simulink model "QC_pid_HIL_control"  (Simulink 7.4)
settings: Solver=ode45  StartTime=0.0  StopTime=inf  RelTol=1e-3
PreLoadFcn:
  | run quadrocopter_param
values from neighbouring files (symbols this model uses):
  phi0 = 0.15    [Quadrocopter_control_Driver.m]    (also in calc_stability.m = 0)
  r_phi0 = 0    [Quadrocopter_control_Driver.m]    (also in calc_stability.m)
  r_psi0 = 0    [Quadrocopter_control_Driver.m]    (also in calc_stability.m)
  r_theta0 = 0    [Quadrocopter_control_Driver.m]    (also in calc_stability.m)
  theta0 = 0.15    [Quadrocopter_control_Driver.m]    (also in calc_stability.m = 0)
  Ts = 0.01    [Reglerauslegung.m]    (also in Test_Reglerauslegung.m)
undefined symbols (not defined in the file or in its folder): boom, f1, f2, f3, f4, f5, g, I_x, I_y, I_z, m
libraries: Copter_Library x6, simulink x4, Control_lib x2
CloseFcn:
  | rtwprivate ssgensfun ModelCloseRequest QC_pid_HIL_control
settings Model: Creator=roczit00  LastModifiedBy=dsatikid

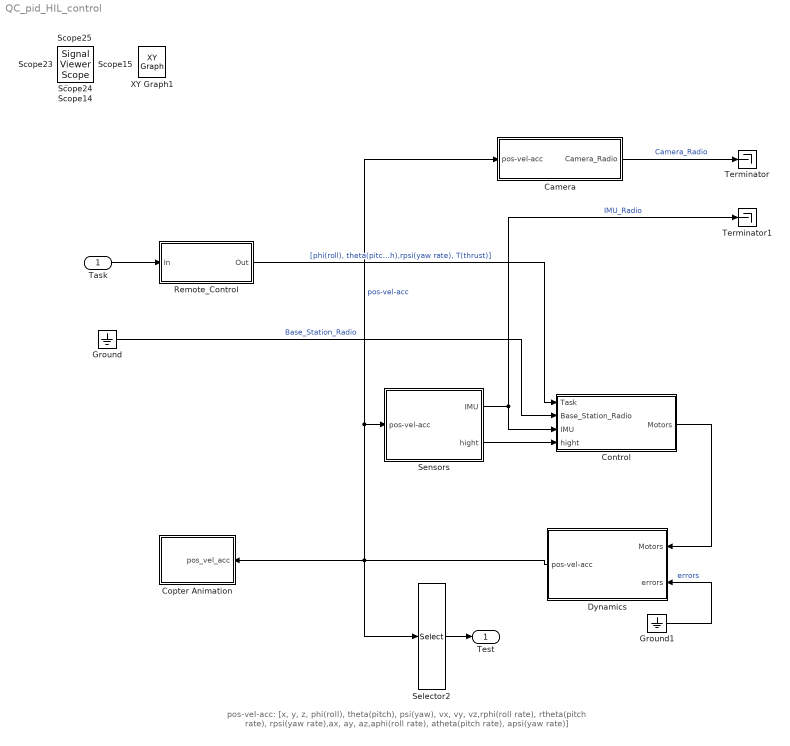
== system QC_pid_HIL_control ==
  note: pos-vel-acc: [x, y, z, phi(roll), theta(pitch), psi(yaw), vx, vy, vz,rphi(roll rate), rtheta(pitch rate), rpsi(yaw rate),ax, ay, az,aphi(roll rate), atheta(pitch rate), apsi(yaw rate)]
  Task : Inport  PortDimensions=4  OutDataType=fixdt(1, 16)  OutScaling=2^0
  Camera : Subsystem
  Control : Subsystem
  Copter Animation : Subsystem  mask(Quadrocopter Animation){AXES=[-100 100 -100 100 0 100], T_INT=1/25, K_VAR=Feste Position, K_POS=[10 0 2], K_ANGLE=27, A_ON=on, u_phi=on, u_theta=on, u_psi=on, u_x=on, u_y=on, u_z=off}
      mask prompts: AXES "Achsen Grenzen [xmin xmax ymin ymax zmin zmax]"; T_INT "Zeitintervall zwischen Aktualisierungen [s]:"; K_VAR "Kamera Art:"; K_POS "Ort der Kamera [xc yc zc]:"; K_ANGLE "Öffnungswinkel der Kamera [Grad]:"; A_ON "Animation Einschalten:"; u_phi "Use Input phi:"; u_theta "Use Input theta:"; u_psi "Use Input psi:"; u_x "Use Input x:"; u_y "Use Input y:"; u_z "Use Input z:"
      mask help: Erstellt eine 3-D animierte Ansicht eines Quadrocopters.
      mask init:
      | Config.axes = AXES;
      | Config.update = T_INT;
      | Config.camera_view = K_VAR;
      | Config.camera_pos = K_POS;
      | Config.view = K_ANGLE;
      | Config.Animenable = A_ON;
      | Config.phi = u_phi;
      | Config.theta = u_theta;
      | Config.psi = u_psi;
      | Config.x = u_x;
      | Config.y = u_y;
      | Config.z = u_z;
      mask Help:
      | <p>Dieser Block erstellt ein 3 dimensionales Fenster eines Quadrocopters.
      | 
      | <p><H4>Block Eingänge</H4>
      | Der Eingangsvektor bestehend aus:
      | <ul>
      | <li>X-Koordinate - Ort bezogen auf die X-Achse
      | <li>Y-Koordinate - Ort bezogen auf die Y-Achse
      | <li>Z-Koordinate - Ort bezogen auf die Z-Achse
      | <li>Psi - Yaw Drehung um die Z-Achse
      | <li>Phi - Roll Drehen um die Achse in Flugrichtung
      | <li>theta - pitch Neigung in Flugrichtung nach oben bzw. unten
      | </ul></p>
      mask StyleString: edit,edit,popup(Feste Position|Frei bewegbar),edit,edit,checkbox,checkbox,checkbox,checkbox,checkbox,checkbox,checkbox
  Dynamics : Subsystem
  Ground : Ground
  Ground1 : Ground
  Remote_Control : Subsystem
  Selector2 : Selector  InputPortWidth=19  IndexOptions=Index vector (dialog)  Indices=[4 5 6]  OutputSizes=1
  Sensors : Subsystem
  Terminator : Terminator
  Terminator1 : Terminator
  Test : Outport  OutDataType=fixdt(1, 16)  OutScaling=2^0
  Scope : SignalViewerScope  IOType=viewer  RefreshTime=0.035000
      settings: YMin=-12500  YMax=22500
  Scope11 : SignalViewerScope  IOType=viewer  LegendLocations="247.3333           139            72      20.33333"  RefreshTime=0.103216
      settings: ShowLegends=on  YMin=-1  YMax=0.75  SaveName=ScopeData11
  Scope14 : SignalViewerScope  IOType=viewer  ZoomMode=yonly  LegendLocations="236.3333           142            82      20.33333"  RefreshTime=0.148000
      settings: ShowLegends=on  YMin=-0.2  YMax=0.8  SaveName=ScopeData14
  Scope15 : SignalViewerScope  IOType=viewer  ZoomMode=yonly  LegendLocations="245.3333           139            74      20.33333"  RefreshTime=0.035000
      settings: ShowLegends=on  YMin=-50  YMax=30  SaveName=ScopeData15
  Scope23 : SignalViewerScope  IOType=viewer  LegendLocations="230.3333           178            71      20.33333"  RefreshTime=0.035000
      settings: ShowLegends=on  YMin=-2  YMax=0.25  SaveName=ScopeData23
  Scope24 : SignalViewerScope  IOType=viewer  LegendLocations="248.3333           141            75      20.33333"  RefreshTime=0.035000
      settings: ShowLegends=on  YMin=-0.3  YMax=0.3  SaveName=ScopeData24
  Scope25 : SignalViewerScope  IOType=viewer  LegendLocations="224.3333           129            85      25.33333"  RefreshTime=0.035000
      settings: ShowLegends=on  YMin=-0.05  YMax=0.175  SaveName=ScopeData25
  XY Graph1 : simulink/Sinks/XY Graph  IOType=viewer  SystemSampleTime=-1  xmin=-50  xmax=50  ymin=-50  ymax=50  st=Ts
  wires:
  Sensors/1(IMU) -> Terminator1/1, Control/3(IMU)  "IMU_Radio"
  Sensors/2(hight) -> Control/4(hight)
  Ground1/1 -> Dynamics/2(errors)  "errors"
  Control/1(Motors) -> Dynamics/1(Motors)
  Dynamics/1(pos-vel-acc) -> Sensors/1(pos-vel-acc), Camera/1(pos-vel-acc), Selector2/1, Copter Animation/1(pos_vel_acc)  "pos-vel-acc"
  Camera/1(Camera_Radio) -> Terminator/1  "Camera_Radio"
  Ground/1 -> Control/2(Base_Station_Radio)  "Base_Station_Radio"
  Remote_Control/1(Out) -> Control/1(Task)  "[phi(roll), theta(pitch),rpsi(yaw rate), T(thrust)]"
  Selector2/1 -> Test/1
  Task/1 -> Remote_Control/1(In)

== system QC_pid_HIL_control/Camera ==
  pos-vel-acc : Inport  OutDataType=fixdt(1, 16)  OutScaling=2^0
  Camera_Radio : Outport  OutDataType=fixdt(1, 16)  OutScaling=2^0
  wires:
  pos-vel-acc/1 -> Camera_Radio/1

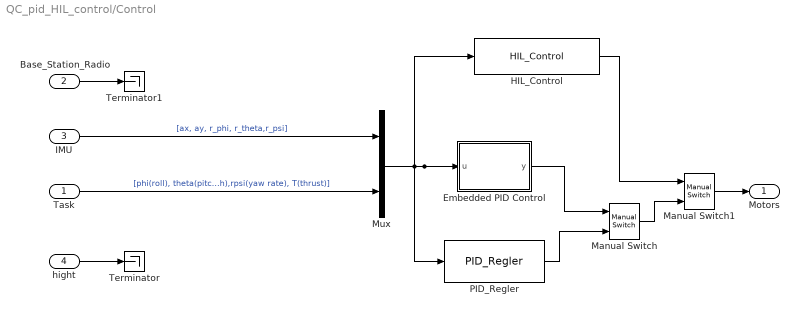
== system QC_pid_HIL_control/Control ==
  Task : Inport  PortDimensions=4  DataType=double  OutDataType=fixdt(1, 16)  OutScaling=2^0  OutDataTypeStr=double
  Base_Station_Radio : Inport  Port=2  OutDataType=fixdt(1, 16)  OutScaling=2^0
  IMU : Inport  Port=3  OutDataType=fixdt(1, 16)  OutScaling=2^0
  hight : Inport  Port=4  DataType=int16  OutDataType=fixdt(1, 16)  OutScaling=2^0  OutDataTypeStr=int16
  Embedded PID Control : Stateflow chart
  HIL_Control : Control_lib/HIL_Control  enabled=on
  Manual Switch : simulink/Signal Routing/Manual Switch  SystemSampleTime=-1  sw=0  action=0  varsize=off
  Manual Switch1 : simulink/Signal Routing/Manual Switch  SystemSampleTime=-1  sw=1  action=0  varsize=off
  Mux : Mux  Inputs=2
  PID_Regler : Control_lib/PID_Regler  SystemSampleTime=-1
  Terminator : Terminator
  Terminator1 : Terminator
  Motors : Outport  PortDimensions=4  OutDataType=fixdt(1, 16)  OutScaling=2^0
  wires:
  Base_Station_Radio/1 -> Terminator1/1
  hight/1 -> Terminator/1
  Mux/1 -> PID_Regler/1, HIL_Control/1, Embedded PID Control/1(u)
  IMU/1 -> Mux/1  "[ax, ay, r_phi, r_theta,r_psi]"
  PID_Regler/1 -> Manual Switch/2
  Task/1 -> Mux/2  "[phi(roll), theta(pitch),rpsi(yaw rate), T(thrust)]"
  Embedded PID Control/1(y) -> Manual Switch/1
  HIL_Control/1 -> Manual Switch1/1
  Manual Switch/1 -> Manual Switch1/2
  Manual Switch1/1 -> Motors/1

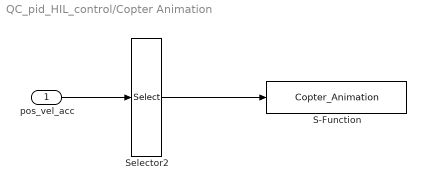
== system QC_pid_HIL_control/Copter Animation ==
  pos_vel_acc : Inport  PortDimensions=19  OutDataType=sfix(16)  OutScaling=2^0
  S-Function : S-Function  FunctionName=Copter_Animation  Parameters=Config  EnableBusSupport=off
  Selector2 : Selector  InputPortWidth=19  IndexOptions=Index vector (dialog)  Indices=[1 2 3 4 5 6]  OutputSizes=1
  wires:
  pos_vel_acc/1 -> Selector2/1
  Selector2/1 -> S-Function/1

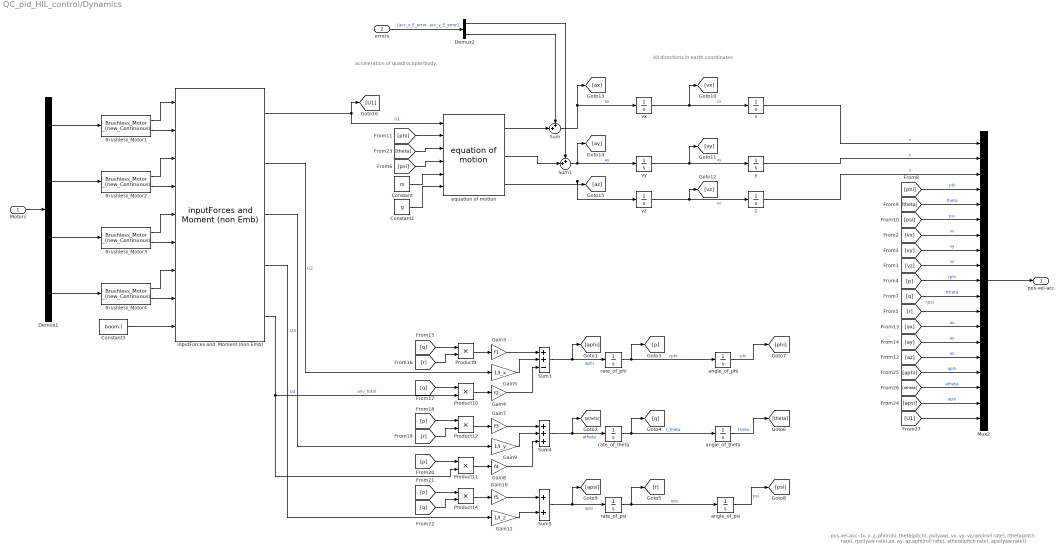
== system QC_pid_HIL_control/Dynamics ==
  note: rpsi
  note: pos-vel-acc: [x, y, z, phi(roll), theta(pitch), psi(yaw), vx, vy, vz,rphi(roll rate), rtheta(pitch rate), rpsi(yaw rate),ax, ay, az,aphi(roll rate), atheta(pitch rate), apsi(yaw rate)]
  note: All directions in earth coordinates
  note: acceleration of quadrocopterbody
  Motors : Inport  OutDataType=fixdt(1, 16)  OutScaling=2^0
  errors : Inport  Port=2  OutDataType=fixdt(1, 16)  OutScaling=2^0
  Brushless_Motor1 : Copter_Library/Brushless_Motor _(new_Continuous)  SystemSampleTime=-1  M_error=1.01
  Brushless_Motor2 : Copter_Library/Brushless_Motor _(new_Continuous)  SystemSampleTime=-1  M_error=1.02
  Brushless_Motor3 : Copter_Library/Brushless_Motor _(new_Continuous)  SystemSampleTime=-1  M_error=0.98
  Brushless_Motor4 : Copter_Library/Brushless_Motor _(new_Continuous)  SystemSampleTime=-1  M_error=0.99
  Constant : Constant  Value=m  OutDataType=fixdt(1, 16)  OutScaling=2^0
  Constant1 : Constant  Value=g  OutDataType=fixdt(1, 16)  OutScaling=2^0
  Constant3 : Constant  Value=boom.l  OutDataType=fixdt(1, 16)  OutScaling=2^0
  Demux1 : Demux
  Demux2 : Demux  Outputs=2
  Gain10 : Gain  Gain=f5  ParameterDataType=fixdt(1, 16)  ParameterScaling=2^0  OutDataType=fixdt(1, 16)  OutScaling=2^0
  Gain12 : Gain  Gain=1/I_z  ParameterDataType=fixdt(1, 16)  ParameterScaling=2^0  OutDataType=fixdt(1, 16)  OutScaling=2^0
  Gain3 : Gain  Gain=f1  ParameterDataType=fixdt(1, 16)  ParameterScaling=2^0  OutDataType=fixdt(1, 16)  OutScaling=2^0
  Gain4 : Gain  Gain=f2  ParameterDataType=fixdt(1, 16)  ParameterScaling=2^0  OutDataType=fixdt(1, 16)  OutScaling=2^0
  Gain5 : Gain  Gain=1/I_x  ParameterDataType=fixdt(1, 16)  ParameterScaling=2^0  OutDataType=fixdt(1, 16)  OutScaling=2^0
  Gain7 : Gain  Gain=f3  ParameterDataType=fixdt(1, 16)  ParameterScaling=2^0  OutDataType=fixdt(1, 16)  OutScaling=2^0
  Gain8 : Gain  Gain=f4  ParameterDataType=fixdt(1, 16)  ParameterScaling=2^0  OutDataType=fixdt(1, 16)  OutScaling=2^0
  Gain9 : Gain  Gain=1/I_y  ParameterDataType=fixdt(1, 16)  ParameterScaling=2^0  OutDataType=fixdt(1, 16)  OutScaling=2^0
  Mux2 : Mux  Inputs=19
  Product{9..12,14} (5 alike) : Product  OutDataType=fixdt(1, 16)  OutScaling=2^0  RndMeth=Zero
  Sum : Sum  Inputs=++|  OutDataType=fixdt(1, 16)  OutScaling=2^0
  Sum1 : Sum  Inputs=++|  OutDataType=fixdt(1, 16)  OutScaling=2^0
  Sum3 : Sum  Inputs=++-  OutDataType=fixdt(1, 16)  OutScaling=2^0
  Sum4 : Sum  Inputs=+++  OutDataType=fixdt(1, 16)  OutScaling=2^0
  Sum5 : Sum  OutDataType=fixdt(1, 16)  OutScaling=2^0
  angle_of_phi : Integrator  InitialCondition=phi0
  angle_of_psi : Integrator
  angle_of_theta : Integrator  InitialCondition=theta0
  equation of motion : Copter_Library/equation of motion  SystemSampleTime=-1
  inputForces and  Moment (non Emb) : Copter_Library/inputForces and  Moment (non Emb)  SystemSampleTime=-1
  rate_of_phi : Integrator  InitialCondition=r_phi0
  rate_of_psi : Integrator  InitialCondition=r_psi0
  rate_of_theta : Integrator  InitialCondition=r_theta0
  vx : Integrator
  vy : Integrator
  vz : Integrator
  x : Integrator
  y : Integrator
  z : Integrator
  pos-vel-acc : Outport  OutDataType=fixdt(1, 16)  OutScaling=2^0
  wires:
  [apsi] -> Mux2/18  "apsi"
  [atheta] -> Mux2/17  "atheta"
  [aphi] -> Mux2/16  "aphi"
  [az] -> Mux2/15  "az"
  [ay] -> Mux2/14  "ay"
  [ax] -> Mux2/13  "ax"
  [r] -> Mux2/12
  [q] -> Mux2/11  "rtheta"
  [p] -> Mux2/10  "rphi"
  [vz] -> Mux2/9  "vz"
  [vy] -> Mux2/8  "vy"
  [vx] -> Mux2/7  "vx"
  [psi] -> Mux2/6  "psi"
  [theta] -> Mux2/5  "theta"
  [phi] -> Mux2/4  "phi"
  z/1 -> Mux2/3  "z"
  Mux2/1 -> pos-vel-acc/1
  errors/1 -> Demux2/1  "[acc_x_E_error, acc_y_E_error]"
  Motors/1 -> Demux1/1
  Demux1/3 -> Brushless_Motor3/1
  Demux1/4 -> Brushless_Motor4/1
  Demux1/2 -> Brushless_Motor2/1
  Demux1/1 -> Brushless_Motor1/1
  vx/1 -> [vx], x/1  "vx"
  vy/1 -> [vy], y/1  "vy"
  vz/1 -> [vz], z/1  "vz"
  Constant3/1 -> inputForces and  Moment (non Emb)/9
  Sum5/1 -> [apsi], rate_of_psi/1  "apsi"
  inputForces and  Moment (non Emb)/4 -> Gain12/1  "U4"
  Gain12/1 -> Sum5/2
  Gain10/1 -> Sum5/1
  Product14/1 -> Gain10/1
  [q] -> Product14/2
  [p] -> Product14/1
  Sum4/1 -> [atheta], rate_of_theta/1  "atheta"
  inputForces and  Moment (non Emb)/3 -> Gain9/1  "U3"
  Gain8/1 -> Sum4/3
  Gain9/1 -> Sum4/2
  Product11/1 -> Gain8/1
  [p] -> Product11/1
  Gain7/1 -> Sum4/1
  Product12/1 -> Gain7/1
  [r] -> Product12/2
  [p] -> Product12/1
  Sum3/1 -> [aphi], rate_of_phi/1  "aphi"
  Gain4/1 -> Sum3/3
  Gain5/1 -> Sum3/2
  inputForces and  Moment (non Emb)/2 -> Gain5/1  "U2"
  Product10/1 -> Gain4/1
  [q] -> Product10/1
  Gain3/1 -> Sum3/1
  Product9/1 -> Gain3/1
  [r] -> Product9/2
  [q] -> Product9/1
  inputForces and  Moment (non Emb)/5 -> Product11/2, Product10/2  "anv_total"
  angle_of_phi/1 -> [phi]  "phi"
  angle_of_theta/1 -> [theta]  "theta"
  angle_of_psi/1 -> [psi]  "psi"
  rate_of_phi/1 -> [p], angle_of_phi/1  "rphi"
  rate_of_theta/1 -> angle_of_theta/1, [q]  "r_theta"
  rate_of_psi/1 -> angle_of_psi/1, [r]  "rpsi"
  Brushless_Motor1/1 -> inputForces and  Moment (non Emb)/1
  Brushless_Motor1/2 -> inputForces and  Moment (non Emb)/2
  Brushless_Motor2/1 -> inputForces and  Moment (non Emb)/3
  Brushless_Motor2/2 -> inputForces and  Moment (non Emb)/4
  Brushless_Motor3/1 -> inputForces and  Moment (non Emb)/5
  Brushless_Motor3/2 -> inputForces and  Moment (non Emb)/6
  Brushless_Motor4/1 -> inputForces and  Moment (non Emb)/7
  Brushless_Motor4/2 -> inputForces and  Moment (non Emb)/8
  x/1 -> Mux2/1  "x"
  y/1 -> Mux2/2  "y"
  Sum1/1 -> [ay], vy/1  "ay"
  Sum/1 -> [ax], vx/1  "ax"
  Demux2/2 -> Sum/1
  Demux2/1 -> Sum1/1
  equation of motion/3 -> [az], vz/1
  equation of motion/2 -> Sum1/2
  equation of motion/1 -> Sum/2
  inputForces and  Moment (non Emb)/1 -> equation of motion/1, [U1]  "U1"
  [phi] -> equation of motion/2
  [theta] -> equation of motion/3
  [psi] -> equation of motion/4
  Constant/1 -> equation of motion/5
  Constant1/1 -> equation of motion/6
  [U1] -> Mux2/19

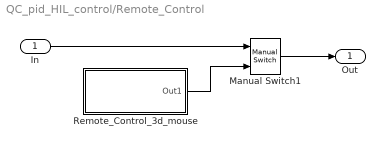
== system QC_pid_HIL_control/Remote_Control ==
  In : Inport  OutDataType=fixdt(1, 16)  OutScaling=2^0
  Manual Switch1 : simulink/Signal Routing/Manual Switch  SystemSampleTime=-1  sw=0  action=0  varsize=off
  Remote_Control_3d_mouse : Subsystem  AncestorBlock=Remote_Control_Library/Remote_Control_3d_mouse
  Out : Outport  OutDataType=fixdt(1, 16)  OutScaling=2^0
  wires:
  In/1 -> Manual Switch1/1
  Manual Switch1/1 -> Out/1
  Remote_Control_3d_mouse/1(Out1) -> Manual Switch1/2

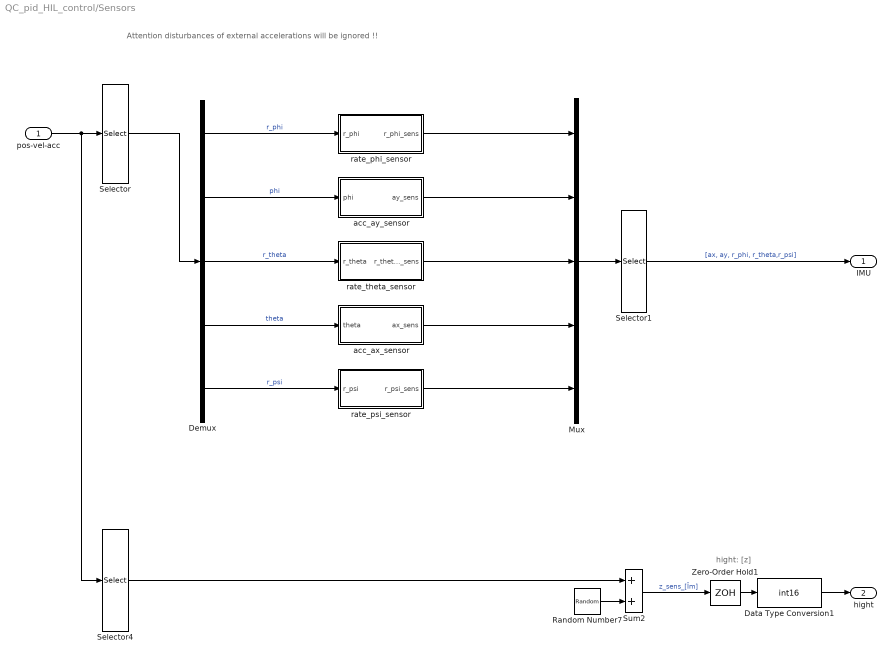
== system QC_pid_HIL_control/Sensors ==
  note: hight: [z]
  note: Attention disturbances of external accelerations will be ignored !!
  pos-vel-acc : Inport  PortDimensions=19  OutDataType=fixdt(1, 16)  OutScaling=2^0
  Data Type Conversion1 : DataTypeConversion  OutDataTypeMode=int16  OutDataType=fixdt(1, 16)  OutScaling=2^0  OutDataTypeStr=int16  RndMeth=Round
  Demux : Demux  Outputs=5
  Mux : Mux  Inputs=5
  Random Number7 : RandomNumber  Variance=0  SampleTime=Ts
  Selector : Selector  InputPortWidth=19  IndexOptions=Index vector (dialog)  Indices=[10 4 11 5 12]  OutputSizes=1
  Selector1 : Selector  InputPortWidth=5  IndexOptions=Index vector (dialog)  Indices=[4 2 1 3 5]  OutputSizes=1
  Selector4 : Selector  InputPortWidth=19  IndexOptions=Index vector (dialog)  Indices=[3]  OutputSizes=1
  Sum2 : Sum  OutDataType=fixdt(1, 16)  OutScaling=2^0
  Zero-Order Hold1 : ZeroOrderHold  SampleTime=Ts
  acc_ax_sensor : Subsystem
  acc_ay_sensor : Subsystem
  rate_phi_sensor : Subsystem
  rate_psi_sensor : Subsystem
  rate_theta_sensor : Subsystem
  IMU : Outport  OutDataType=fixdt(1, 16)  OutScaling=2^0
  hight : Outport  Port=2  OutDataType=fixdt(1, 16)  OutScaling=2^0
  wires:
  Random Number7/1 -> Sum2/2
  pos-vel-acc/1 -> Selector/1, Selector4/1
  Selector/1 -> Demux/1
  Selector4/1 -> Sum2/1
  Sum2/1 -> Zero-Order Hold1/1  "z_sens_[Ïm]"
  Zero-Order Hold1/1 -> Data Type Conversion1/1
  Data Type Conversion1/1 -> hight/1
  rate_phi_sensor/1(r_phi_sens) -> Mux/1
  acc_ay_sensor/1(ay_sens) -> Mux/2
  rate_theta_sensor/1(r_theta_sens) -> Mux/3
  acc_ax_sensor/1(ax_sens) -> Mux/4
  rate_psi_sensor/1(r_psi_sens) -> Mux/5
  Demux/1 -> rate_phi_sensor/1(r_phi)  "r_phi"
  Demux/2 -> acc_ay_sensor/1(phi)  "phi"
  Demux/3 -> rate_theta_sensor/1(r_theta)  "r_theta"
  Demux/4 -> acc_ax_sensor/1(theta)  "theta"
  Demux/5 -> rate_psi_sensor/1(r_psi)  "r_psi"
  Mux/1 -> Selector1/1
  Selector1/1 -> IMU/1  "[ax, ay, r_phi, r_theta,r_psi]"

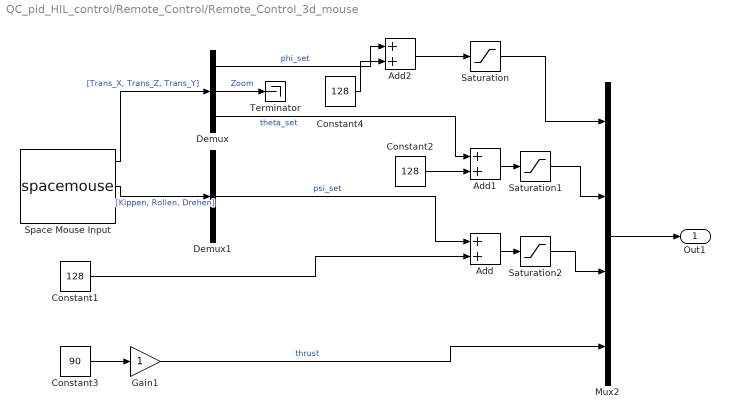
== system QC_pid_HIL_control/Remote_Control/Remote_Control_3d_mouse ==
  Add : Sum  OutDataType=fixdt(1, 16)  OutScaling=2^-10
  Add1 : Sum  OutDataType=fixdt(1, 16)  OutScaling=2^-10
  Add2 : Sum  OutDataType=fixdt(1, 16)  OutScaling=2^-10
  Constant1 : Constant  Value=128  OutDataType=fixdt(1, 16)  OutScaling=2^0
  Constant2 : Constant  Value=128  OutDataType=fixdt(1, 16)  OutScaling=2^0
  Constant3 : Constant  Value=90  OutDataType=fixdt(1, 16)  OutScaling=2^0
  Constant4 : Constant  Value=128  OutDataType=fixdt(1, 16)  OutScaling=2^0
  Demux : Demux  Outputs=3
  Demux1 : Demux  Outputs=3
  Gain1 : Gain  ParameterDataType=fixdt(1, 16)  ParameterScaling=2^0  OutDataType=fixdt(1, 16)  OutScaling=2^0
  Mux2 : Mux
  Saturation : Saturate  UpperLimit=255  LowerLimit=0  OutDataType=fixdt(1, 16)  OutScaling=2^0
  Saturation1 : Saturate  UpperLimit=255  LowerLimit=0  OutDataType=fixdt(1, 16)  OutScaling=2^0
  Saturation2 : Saturate  UpperLimit=255  LowerLimit=0  OutDataType=fixdt(1, 16)  OutScaling=2^0
  Space Mouse Input : S-Function  AncestorBlock=vrlib/Space Mouse Input  FunctionName=spacemouse  Parameters=Port, OutputType, InitialPosition, InitialRotation, PositionSensitivity, RotationSensitivity, Dominant, NormalizeAngle, DisableTranslation, DisableRotation, PositionLow, PositionUp, EnableLimit  EnableBusSupport=off  mask(Space Mouse Input){Port=USB1, OutputType=Speed, Dominant=off, DisableTranslation=off, DisableRotation=off, NormalizeAngle=off, EnableLimit=on, PositionSensitivity=15, RotationSensitivity=15, InitialPosition=[0 0 0], InitialRotation=[0 0 0], PositionLow=[0 0 0], PositionUp=[255 255 255]}
      mask prompts: OutputType "Output type:"; Dominant "Dominant mode"; DisableTranslation "Disable position movement"; DisableRotation "Disable rotation movement"; NormalizeAngle "Normalize output angle"; EnableLimit "Limit position"; PositionSensitivity "Position sensitivity:"; RotationSensitivity "Rotation sensitivity:"; InitialPosition "Initial position:"; InitialRotation "Initial rotation:"; PositionLow "Lower position limit:"; PositionUp "Upper position limit:"
      mask help: Space Mouse input device driver.
      mask Help: helpview(fullfile(docroot, 'toolbox', 'sl3d', 'sl3d.map'), 'vr_magellanspacemouse');
      mask StyleString: popup(COM1|COM2|COM3|COM4|USB1|USB2|USB3|USB4|USB),popup(Speed|Position|Viewpoint coordinates),checkbox,checkbox,checkbox,checkbox,checkbox,edit,edit,edit,edit,edit,edit
      mask CallbackString: spacemousemask|spacemousemask|||||spacemousemask||||||
      mask Display:
      | image(imread('spacemouseicon.png'))
      | port_label('output', 1, 'Translation')
      | port_label('output', 2, 'Rotation')
      | port_label('output', 3, 'Buttons')
  Terminator : Terminator
  Out1 : Outport  OutDataType=fixdt(1, 16)  OutScaling=2^0
  wires:
  Demux/1 -> Add2/1  "phi_set"
  Constant4/1 -> Add2/2
  Demux/3 -> Add1/1  "theta_set"
  Constant2/1 -> Add1/2
  Add/1 -> Saturation2/1
  Demux1/2 -> Add/1  "psi_set"
  Constant1/1 -> Add/2
  Space Mouse Input/2 -> Demux1/1  "[Kippen, Rollen, Drehen]"
  Demux/2 -> Terminator/1  "Zoom"
  Space Mouse Input/1 -> Demux/1  "[Trans_X, Trans_Z, Trans_Y]"
  Constant3/1 -> Gain1/1
  Gain1/1 -> Mux2/4  "thrust"
  Mux2/1 -> Out1/1
  Add2/1 -> Saturation/1
  Add1/1 -> Saturation1/1
  Saturation1/1 -> Mux2/2
  Saturation2/1 -> Mux2/3
  Saturation/1 -> Mux2/1

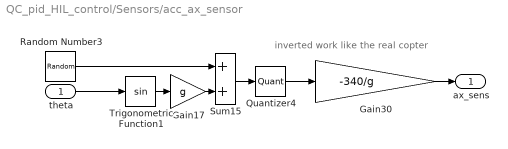
== system QC_pid_HIL_control/Sensors/acc_ax_sensor ==
  note: inverted work like the real copter
  theta : Inport  OutDataType=fixdt(1, 16)  OutScaling=2^0
  Gain17 : Gain  Gain=g  ParameterDataType=fixdt(1, 16)  ParameterScaling=2^0  OutDataType=fixdt(1, 16)  OutScaling=2^0
  Gain30 : Gain  Gain=-340/g  ParameterDataType=fixdt(1, 16)  ParameterScaling=2^0  OutDataType=fixdt(1, 16)  OutScaling=2^0
  Quantizer4 : Quantizer  QuantizationInterval=g/340  SampleTime=Ts
  Random Number3 : RandomNumber  Variance=0.0003  Seed=676  SampleTime=Ts
  Sum15 : Sum  OutDataType=fixdt(1, 16)  OutScaling=2^0
  Trigonometric Function1 : Trigonometry
  ax_sens : Outport  OutDataType=fixdt(1, 16)  OutScaling=2^0
  wires:
  Random Number3/1 -> Sum15/1
  Sum15/1 -> Quantizer4/1
  Trigonometric Function1/1 -> Gain17/1
  Gain17/1 -> Sum15/2
  Quantizer4/1 -> Gain30/1
  theta/1 -> Trigonometric Function1/1
  Gain30/1 -> ax_sens/1

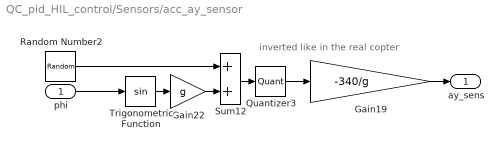
== system QC_pid_HIL_control/Sensors/acc_ay_sensor ==
  note: inverted like in the real copter
  phi : Inport  OutDataType=fixdt(1, 16)  OutScaling=2^0
  Gain19 : Gain  Gain=-340/g  ParameterDataType=fixdt(1, 16)  ParameterScaling=2^0  OutDataType=fixdt(1, 16)  OutScaling=2^0
  Gain22 : Gain  Gain=g  ParameterDataType=fixdt(1, 16)  ParameterScaling=2^0  OutDataType=fixdt(1, 16)  OutScaling=2^0
  Quantizer3 : Quantizer  QuantizationInterval=g/340  SampleTime=Ts
  Random Number2 : RandomNumber  Variance=0.0003  Seed=4564  SampleTime=0.01
  Sum12 : Sum  OutDataType=fixdt(1, 16)  OutScaling=2^0
  Trigonometric Function : Trigonometry
  ay_sens : Outport  OutDataType=fixdt(1, 16)  OutScaling=2^0
  wires:
  Random Number2/1 -> Sum12/1
  Sum12/1 -> Quantizer3/1
  Trigonometric Function/1 -> Gain22/1
  Gain22/1 -> Sum12/2
  Quantizer3/1 -> Gain19/1
  phi/1 -> Trigonometric Function/1
  Gain19/1 -> ay_sens/1

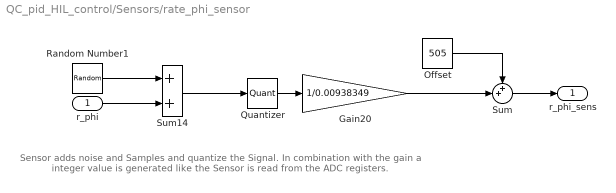
== system QC_pid_HIL_control/Sensors/rate_phi_sensor ==
  note: Sensor adds noise and Samples and quantize the Signal. In combination with the gain a integer value is generated
      | like the Sensor is read from the ADC registers.
  r_phi : Inport  OutDataType=fixdt(1, 16)  OutScaling=2^0
  Gain20 : Gain  Gain=1/0.00938349  ParameterDataType=fixdt(1, 16)  ParameterScaling=2^0  OutDataType=fixdt(1, 16)  OutScaling=2^0
  Offset : Constant  Value=505  OutDataType=fixdt(1, 16)  OutScaling=2^0
  Quantizer : Quantizer  QuantizationInterval=0.00938349  SampleTime=Ts
  Random Number1 : RandomNumber  Variance=3.0462e-8  Seed=45632  SampleTime=0.01
  Sum : Sum  Inputs=++|  OutDataType=fixdt(1, 16)  OutScaling=2^0
  Sum14 : Sum  OutDataType=fixdt(1, 16)  OutScaling=2^0
  r_phi_sens : Outport  OutDataType=fixdt(1, 16)  OutScaling=2^0
  wires:
  Random Number1/1 -> Sum14/1
  Sum14/1 -> Quantizer/1
  Quantizer/1 -> Gain20/1
  r_phi/1 -> Sum14/2
  Gain20/1 -> Sum/2
  Offset/1 -> Sum/1
  Sum/1 -> r_phi_sens/1

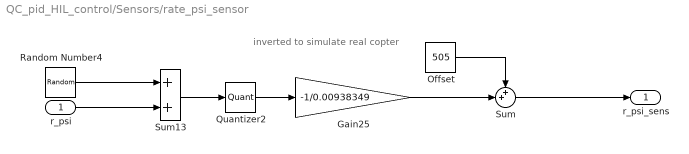
== system QC_pid_HIL_control/Sensors/rate_psi_sensor ==
  note: inverted to simulate real copter
  r_psi : Inport  OutDataType=fixdt(1, 16)  OutScaling=2^0
  Gain25 : Gain  Gain=-1/0.00938349  ParameterDataType=fixdt(1, 16)  ParameterScaling=2^0  OutDataType=fixdt(1, 16)  OutScaling=2^0
  Offset : Constant  Value=505  OutDataType=fixdt(1, 16)  OutScaling=2^0
  Quantizer2 : Quantizer  QuantizationInterval=0.00938349  SampleTime=Ts
  Random Number4 : RandomNumber  Variance=3.0462e-8  Seed=1634  SampleTime=0.01
  Sum : Sum  Inputs=++|  OutDataType=fixdt(1, 16)  OutScaling=2^0
  Sum13 : Sum  OutDataType=fixdt(1, 16)  OutScaling=2^0
  r_psi_sens : Outport  OutDataType=fixdt(1, 16)  OutScaling=2^0
  wires:
  Random Number4/1 -> Sum13/1
  Sum13/1 -> Quantizer2/1
  Quantizer2/1 -> Gain25/1
  r_psi/1 -> Sum13/2
  Offset/1 -> Sum/1
  Gain25/1 -> Sum/2
  Sum/1 -> r_psi_sens/1

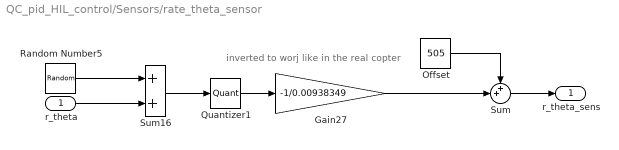
== system QC_pid_HIL_control/Sensors/rate_theta_sensor ==
  note: inverted to worj like in the real copter
  r_theta : Inport  OutDataType=fixdt(1, 16)  OutScaling=2^0
  Gain27 : Gain  Gain=-1/0.00938349  ParameterDataType=fixdt(1, 16)  ParameterScaling=2^0  OutDataType=fixdt(1, 16)  OutScaling=2^0
  Offset : Constant  Value=505  OutDataType=fixdt(1, 16)  OutScaling=2^0
  Quantizer1 : Quantizer  QuantizationInterval=0.00938349  SampleTime=Ts
  Random Number5 : RandomNumber  Variance=3.0462e-8  Seed=4731  SampleTime=0.01
  Sum : Sum  Inputs=++|  OutDataType=fixdt(1, 16)  OutScaling=2^0
  Sum16 : Sum  OutDataType=fixdt(1, 16)  OutScaling=2^0
  r_theta_sens : Outport  OutDataType=fixdt(1, 16)  OutScaling=2^0
  wires:
  Random Number5/1 -> Sum16/1
  Sum16/1 -> Quantizer1/1
  Quantizer1/1 -> Gain27/1
  r_theta/1 -> Sum16/2
  Offset/1 -> Sum/1
  Gain27/1 -> Sum/2
  Sum/1 -> r_theta_sens/1

== matlab function Control/Embedded PID Control ==
  settings: updateMethod=DISCRETE  sampleTime=0.005
  data: u input double; y output double
function y = fcn(u)
%#eml
persistent e_r_Roll_1 e_Roll_1 r_Roll_I_State r_Roll_Filter_State 
persistent e_r_Pitch_1 e_Pitch_1 r_Pitch_I_State r_Pitch_Filter_State 
persistent e_r_Yaw_1 r_Yaw_I_State r_Yaw_Filter_State
persistent M1_limited M2_limited M3_limited M4_limited 
%  first time initialization
if isempty(M1_limited) 
    M1_limited=uint8(0);
    M2_limited=uint8(0);
    M3_limited=uint8(0);
    M4_limited=uint8(0);
    e_r_Roll_1 = double(0);
    e_Roll_1 = double(0);
    r_Roll_I_State = double(0);
    r_Roll_Filter_State = double(0); 
    e_r_Pitch_1 = double(0);
    e_Pitch_1 = double(0);
    r_Pitch_I_State = double(0); 
    r_Pitch_Filter_State = double(0); 
    e_r_Yaw_1 = double(0); 
    r_Yaw_I_State = double(0); 
    r_Yaw_Filter_State = double(0);
end
IRoll = double(0);
FiltRoll = double(0);
IPitch = double(0);
FiltPitch = double(0);
Ts = 0.005; % sec
G = 9.810; % m/sec²
maxRemotePitch = 128;
maxRemoteRoll = 128;
maxRemoteYaw = 128;
maxPitchAngle = pi/4;
maxRollAngle  = pi/4;
maxYawRate = 200;
sensorSensitivityX = 340;
sensorSensitivityY = 340;
sensorSensitivityZ = 340;
copterState.gyroPOffset = 505;
copterState.gyroROffset = 505;
copterState.gyroYOffset = 505;
copterState.YawRateI_State = 0;
copterState.YawRateD_Filter = 0;
copterState.PitchRateI_State = 0;
copterState.PitchRateD_Filter = 0;
copterState.RollRateI_State = 0;
copterState.RollRateD_Filter = 0;
% copy inputs to variables with easy to know names
copterState.angVelRRaw =  u(3);
copterState.accYRaw = u(2);
copterState.angVelPRaw = u(4);
copterState.accXRaw = u(1);
copterState.accZRaw = 0; %not available
copterState.angVelYRaw = u(5);
copterState.remoteForceRaw = u(9);
copterState.remotePitchRaw = u(7);
copterState.remoteRollRaw = u(6);
copterState.remoteYawRaw = u(8);
copterState.accY = int16(0);
copterState.accX = int16(0);
copterState.accZ = int16(0);
copterState.angP = int16(0);
copterState.angR = int16(0);
copterState.angVelP = int16(0);
copterState.angVelR = int16(0);
copterState.angVelY = int16(0);
copterState.remotePitch = int16(0);
copterState.remoteRoll = int16(0);
copterState.remoteForce = int16(0);
copterState.remoteYaw = int16(0);
angP = double(0);
angR = double(0);

% Convert Data like in the copter
% Accelerometer
%%%%%%%%%%%%%%%%%
  %/* calculate the physical acceleration values in [(10 * m)/(s^2)], as needed by the control algorithm */
  copterState.accY = int16(((int32(copterState.accYRaw) * G) / sensorSensitivityY) / 10);
  copterState.accX = -int16(((int32(copterState.accXRaw) * G) / sensorSensitivityX) / 10);
  copterState.accZ = -int16(((int32(copterState.accZRaw) * G) / sensorSensitivityZ) / 10);
  %// [ 10000*rad ]
  copterState.angP = -int16(int32(copterState.accXRaw)*1000/340);
  copterState.angR = -int16(int32(copterState.accYRaw)*1000/340);
  
  % Gyroscopes [100 * rad/sec]
  %%%%%%%%%%%%%%
   copterState.angVelP     = -int16(double(copterState.angVelPRaw-copterState.gyroPOffset) * 0.938349);
   copterState.angVelR     = int16(double(copterState.angVelRRaw-copterState.gyroROffset) * 0.938349);
   copterState.angVelY     = -int16(double(copterState.angVelYRaw-copterState.gyroYOffset) * 0.938349);
   
   % Remote
   %%%%%%%%%%%%%
  copterState.remotePitch    = int16(maxPitchAngle*int32(copterState.remotePitchRaw-128)/maxRemotePitch);
  copterState.remoteRoll     = -int16(maxRollAngle*int32(copterState.remoteRollRaw-128)/maxRemoteRoll);
  copterState.remoteForce    = int16(copterState.remoteForceRaw); 
  copterState.remoteYaw      = int16(maxYawRate*int32(copterState.remoteYawRaw-128)/maxRemoteYaw);

% Set outputs to Values calculated last sample time
y = double([M1_limited;M2_limited;M3_limited;M4_limited]);
   
   angP = double(copterState.angP)/1000;
   angR = double(copterState.angR)/1000;
   
% calculate error values for the controlled angles
   % Pitch error 
   e_Pitch = double(copterState.remotePitch) - angP;
   % Roll error
   e_Roll = double(copterState.remoteRoll) - angR;
   % calculate controller output for the angles (I State & FilterState are not necessary cause only p is used
   [m_Roll, IRoll, FiltRoll] = PID(150,0.5,0,0,e_Roll,e_Roll_1,IRoll, FiltRoll, Ts);
   [m_Pitch, IPitch, FiltPitch] = PID(150,0.5,0,0,e_Pitch,e_Pitch_1,IPitch,FiltPitch,Ts);
      
   % Yaw Rate error
   e_r_Yaw = double(copterState.remoteYaw) - double(copterState.angVelY);
   % Pitch Rate error
   e_r_Pitch = m_Pitch - double(copterState.angVelP);
   % Roll Rate error
   e_r_Roll = m_Roll - double(copterState.angVelR);
   % calculate  controller output for rates
   [m_r_Yaw,r_Yaw_I_State, r_Yaw_Filter_State] = PID (70, ...
       0.5, 0,0,e_r_Yaw, e_r_Yaw_1, r_Yaw_I_State, r_Yaw_Filter_State,Ts);
   [m_r_Roll,r_Roll_I_State, r_Roll_Filter_State] = PID (70, ...
       0.5, 0,0,e_r_Roll, e_r_Roll_1, r_Roll_I_State, r_Roll_Filter_State,Ts);
   [m_r_Pitch,r_Pitch_I_State, r_Pitch_Filter_State] = PID (70, ...
       0.5, 0,0,e_r_Pitch, e_r_Pitch_1, r_Pitch_I_State, r_Pitch_Filter_State,Ts);
   
   % save error for next sample time
   e_Roll_1 = e_Roll;
   e_Pitch_1 = e_Pitch;
   e_r_Roll_1 = e_r_Roll;
   e_r_Pitch_1 = e_r_Pitch;
   e_r_Yaw_1 = e_r_Yaw;
 
   %//Calculate new setpoints of all motors
    M1 = (copterState.remoteForce-m_r_Pitch+m_r_Yaw);
    M2 = (copterState.remoteForce+m_r_Roll-m_r_Yaw);
    M3 = (copterState.remoteForce+m_r_Pitch+m_r_Yaw);
    M4 = (copterState.remoteForce-m_r_Roll-m_r_Yaw);
   
   
    %// saturate setpoint of motor1 to 0 if less and 255 if above
    if M1 < 0
      M1_limited = uint8(0);
    else
        if M1 > 255
            M1_limited = uint8(255); 
        else
            M1_limited=uint8(M1);
        end
    end
    
    %// saturate setpoint of motor2 to 0 if less and 255 if above
    if M2 < 0
      M2_limited = uint8(0);
    else
        if M2 > 255
          M2_limited = uint8(255); 
        else
          M2_limited=uint8(M2);
        end
    end

    %// saturate setpoint of motor3 to 0 if less and 255 if above
  if M3 < 0
      M3_limited = uint8(0);
  else
      if M3 > 255
        M3_limited = uint8(255); 
      else
         M3_limited=uint8(M3);
      end
  end
    
    %// saturate setpoint of motor4 to 0 if less and 255 if above
    if M4 < 0
      M4_limited = uint8(0);
    else
        if M4 > 255
           M4_limited = uint8(255); 
        else
           M4_limited=uint8(M4);
        end
    end

% This function calculates the next Value of the ?ideal? PID controller
function [ret, I_State, Filt_State] = PID (P, I, D, N, ek, ek_1, I_State, Filt_State, Ts)

if P ~= 0 
    if I ~= 0
        % calculate new itegral value
        I_State = ek * Ts * I + I_State;
    else
        I_State = 0;
    end

    if D ~= 0
        % calculate new derivative Value
        yd = (ek - ek_1)/Ts * D;

        % Filter the derivative  Value
        Filt_State = Ts * (yd -N*Filt_State)+ Filt_State ;
    else
        Filt_State = 0;
    end

    % Add all values and multiply P gain to all
    ret = (P * ek + I_State + Filt_State);

else
    ret = 0;
end


function ret16 = mult_fp (A, B, factor)
    ret32 = int32(A) * int32(B)/factor;
    if ret32 > 2^15-1
        ret16 = int16(2^15-1);
    else
        if ret32 < -2^15+1
            ret16 = int16(-2^15+1);
        else
            ret16 = int16(ret32);
        end
    end
% end of mult_fp    

function ret16 = div_fp(A, B, factor)
if B == 0
    display('divide by ZERO !!!!')
    ret16 = 2^16-1;
else
    ret32 = int32(A)*factor/int32(B);
     if ret32 > 2^15-1
        ret16 = int16(2^15-1);
    else
        if ret32 < -2^15+1
            ret16 = int16(-2^15+1);
        else
            ret16 = int16(ret32);
        end
    end
end
% end of div_fp
